simulink model "subsToComp"  (R2020b)
settings: Solver=FixedStepAuto  StartTime=0.0  StopTime=10.0  FixedStep=1/100000  RelTol=1e-3
libraries: fl_lib x8, nesl_utility x4
settings Model: Creator=i7  LastModifiedBy=i7

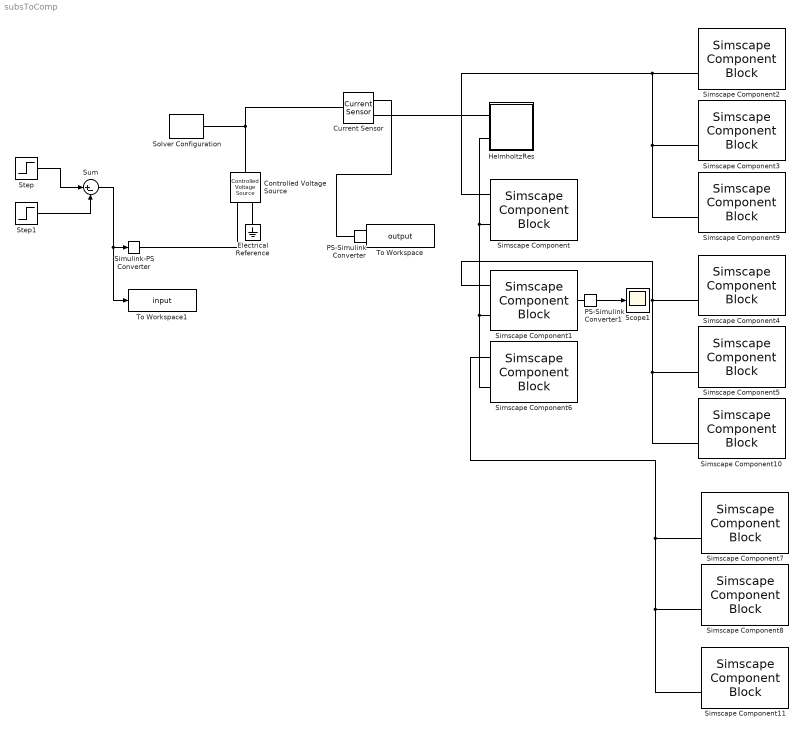
== system subsToComp ==
  Controlled Voltage Source : fl_lib/Electrical/Electrical Sources/Controlled Voltage Source
  Current Sensor : fl_lib/Electrical/Electrical Sensors/Current Sensor
  Electrical Reference : fl_lib/Electrical/Electrical Elements/Electrical Reference
  HelmholtzRes : Subsystem  mask{R=4.116, l=1.2e-3, c=7.08e-07}
      mask prompts: R "Resistance"; l "Inductance"; c "Capacitance"
      mask TypeOptions R: Resistor/R
      mask TypeOptions l: Inductor/l
      mask TypeOptions c: Capacitor/c
  PS-Simulink Converter : nesl_utility/PS-Simulink Converter  PhysicalDomain=network_engine_domain  SubClassName=ps_output  LeftPortType=input  RightPortType=output  PseudoPeriodic=off  Frequencies=[]  Unit=inherit  AffineConversion=off
  PS-Simulink Converter1 : nesl_utility/PS-Simulink Converter  PhysicalDomain=network_engine_domain  SubClassName=ps_output  LeftPortType=input  RightPortType=output  PseudoPeriodic=off  Frequencies=[]  Unit=inherit  AffineConversion=off
  Scope1 : Scope
  Simscape Component{,1..11} (12 alike) : SimscapeComponentBlock  SourceFile=HelmholtzRes  ComponentPath=HelmholtzRes  ComponentVariants="[\"HelmholtzRes\"]"  ComponentVariantNames="[\"HelmholtzRes\"]"  ClassName=HelmholtzRes  SchemaVersion=1  c=7.08e-07 F  l=.0012 H  R=4.116 Ohm
      settings: CopyFcn=simscape.engine.sli.internal.componentblockcallback(gcbh,'COPY')  PreCopyFcn=simscape.engine.sli.internal.componentblockcallback(gcbh,'PRECOPY')  PreDeleteFcn=simscape.engine.sli.internal.componentblockcallback(gcbh,'PREDELETE')  InternalSimscapePortConfiguration="{\"Bottom\":[],\"Left\":[{\"id\":\"out\",\"label\":\"out\",\"type\":\"foundation.electrical.electrical\"},{\"id\":\"in0\",\"label\":\"in0\",\"type\":\"foundation.electrical.electrical\"}],\"Right\":[{\"id\":\"flow\",\"label\":\"flow\",\"type\":\"output\"}],\"Top\":[]}"
      mask Type: HelmholtzRes
  Simulink-PS Converter : nesl_utility/Simulink-PS Converter  PhysicalDomain=network_engine_domain  SubClassName=ps_input  LeftPortType=input  RightPortType=output  PseudoPeriodic=off  Frequencies=[]  NoiseDistribution=none  NoiseParameters=[]  Unit=1  AffineConversion=off  FilteringAndDerivatives=provide  SimscapeFilterOrder=1  InputFilterTimeConstant=0.001  UdotUserProvided=0
  Solver Configuration : nesl_utility/Solver Configuration  PhysicalDomain=network_engine_domain  SubClassName=solver  LeftPortType=input  RightPortType=generic  Tones=[]  Harmonics=[]  SimulateNoise=off  Profile=off  UseLocalSampling=off  EnableSwitchedLinearOptims=on  FrequencyDomain=off  UseCCode=off  RelTol=0.001  AbsTol=1e-06  MinStep=1e-09  ToWorkspace=off  RevertToSquareIcSolve=off  NumHomotopyIterations=100  PhasorMode=off  PhasorModeNumHarmonics=1  DoDC=off  ResidualTolerance=1e-09  UseLocalSolver=off  LocalSolverChoice=NE_BACKWARD_EULER_ADVANCER  LocalSolverSampleTime=0.001  DoFixedCost=off  MaxNonlinIter=3  MaxModeIter=2  ComputeImpulses=off  ImpulseIterations=2  LinearAlgebra=auto  EquationFormulation=NE_TIME_EF  DelaysMemoryBudget=1024  AutomaticFiltering=on  FilteringTimeConstant=0.001  PartitionStorageMethod=AS_NEEDED  PartitionMemoryBudget=1024  PartitionMethod=ROBUST
  Step : Step  SampleTime=0
  Step1 : Step  Time=1 + 1/100000  SampleTime=0
  Sum : Sum  Inputs=|+-
  To Workspace : ToWorkspace  VariableName=output  SaveFormat=Timeseries  SampleTime=-1
  To Workspace1 : ToWorkspace  VariableName=input  SaveFormat=Timeseries  SampleTime=-1
  wires:
  Step/1 -> Sum/1
  Step1/1 -> Sum/2
  Sum/1 -> To Workspace1/1, Simulink-PS Converter/1
  PS-Simulink Converter1/1 -> Scope1/1
  PS-Simulink Converter/1 -> To Workspace/1
  connections:
  Controlled Voltage Source/LConn1 -- Current Sensor/LConn1 -- Solver Configuration/RConn1
  Simulink-PS Converter/RConn1 -- Controlled Voltage Source/RConn1
  Electrical Reference/LConn1 -- Controlled Voltage Source/RConn2
  HelmholtzRes/LConn2 -- Simscape Component6/LConn2 -- Simscape Component1/LConn2 -- Simscape Component/LConn2
  Simscape Component/LConn1 -- Simscape Component9/LConn2 -- Simscape Component3/LConn2 -- Simscape Component2/LConn2
  Simscape Component5/LConn2 -- Simscape Component10/LConn2 -- Simscape Component1/LConn1 -- Simscape Component4/LConn2
  PS-Simulink Converter1/LConn1 -- Simscape Component1/RConn1
  Simscape Component7/LConn2 -- Simscape Component11/LConn2 -- Simscape Component8/LConn2 -- Simscape Component6/LConn1
  Current Sensor/RConn2 -- HelmholtzRes/LConn1
  Current Sensor/RConn1 -- PS-Simulink Converter/LConn1

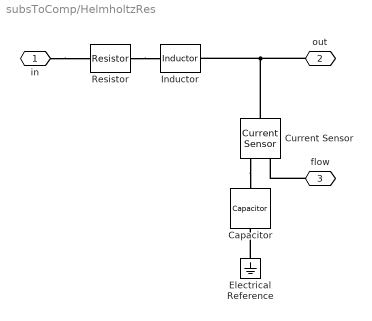
== system subsToComp/HelmholtzRes ==
  Capacitor : fl_lib/Electrical/Electrical Elements/Capacitor  c=c F  r=0 Ohm  g=0 1/Ohm  i_specify=off  i_priority=None  i=0 A  i_nominal_specify=off  i_nominal_unit=A  i_nominal_value=1  v_specify=off  v_priority=None  v=0 V  v_nominal_specify=off  v_nominal_unit=V  v_nominal_value=1  vc_specify=off  vc_priority=High  vc=0 V  vc_nominal_specify=off  vc_nominal_unit=V  vc_nominal_value=1
  Current Sensor : fl_lib/Electrical/Electrical Sensors/Current Sensor
  Electrical Reference : fl_lib/Electrical/Electrical Elements/Electrical Reference
  Inductor : fl_lib/Electrical/Electrical Elements/Inductor  l=l H  r=0 Ohm  g=0 1/Ohm  i_specify=off  i_priority=None  i=0 A  i_nominal_specify=off  i_nominal_unit=A  i_nominal_value=1  v_specify=off  v_priority=None  v=0 V  v_nominal_specify=off  v_nominal_unit=V  v_nominal_value=1  i_L_specify=off  i_L_priority=High  i_L=0 A  i_L_nominal_specify=off  i_L_nominal_unit=A  i_L_nominal_value=1
  Resistor : fl_lib/Electrical/Electrical Elements/Resistor  R=R Ohm  i_specify=off  i_priority=None  i=0 A  i_nominal_specify=off  i_nominal_unit=A  i_nominal_value=1  v_specify=off  v_priority=None  v=0 V  v_nominal_specify=off  v_nominal_unit=V  v_nominal_value=1
  in : PMIOPort  Side=Left
  out : PMIOPort  Port=2  Side=Left
  flow : PMIOPort  Port=3  Side=Right
  connections:
  Electrical Reference/LConn1 -- Capacitor/RConn1
  out/RConn1 -- Current Sensor/LConn1 -- Inductor/RConn1
  in/RConn1 -- Resistor/LConn1
  Resistor/RConn1 -- Inductor/LConn1
  Current Sensor/RConn2 -- Capacitor/LConn1
  flow/RConn1 -- Current Sensor/RConn1
